simulink model "long"  (R2013b)
settings: Solver=ode45  StartTime=0.0  StopTime=10  RelTol=1e-3
values from neighbouring files (symbols this model uses):
  A = [[X_u, X_w, 0, -g*cos(theta_0), 0] ... (first row only)    [hw3.m]
  B = [X_d_e ... (first row only)    [hw3.m]
  C = eye(5)    [hw3.m]
  D = [0; 0; 0; 0; 0]    [hw3.m]
libraries: simulink_extras x6
settings Model: Creator=rjoyce  LastModifiedBy=Johnny
settings DataIOCC: SignalLoggingSaveFormat=ModelDataLogs
settings OptimizationCC: ExpressionDepthLimit=2147483647  SimCompilerOptimization=off
settings DebuggingCC: FcnCallInpInsideContextMsg=UseLocalSettings  FrameProcessingCompatibilityMsg=error  StateNameClashWarn=warning
settings RTWCC: RTWCompilerOptimization=off
settings GRTTargetCC: TargetLangStandard=C89/C90 (ANSI)  CodeReplacementLibrary=None  CombineOutputUpdateFcns=off  CPPClassGenCompliant=on  GRTInterface=on

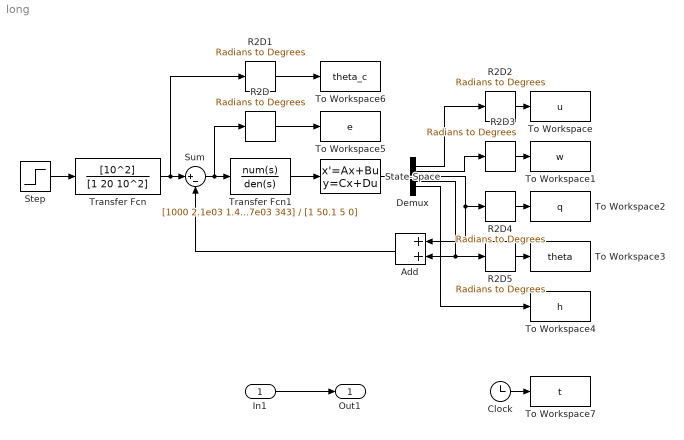
== system long ==
  In1 : Inport
  Add : Sum
  Clock : Clock
  Demux : Demux  Outputs=5
  R2D{,1..5} (6 alike) : simulink_extras/Transformations/Radians to Degrees
  State-Space : StateSpace  A=A  B=B  C=C  D=D  X0=[0 0 0 0 0]
  Step : Step  Time=0  After=5/57.3  SampleTime=0
  Sum : Sum  Inputs=|+-
  To Workspace : ToWorkspace  VariableName=u  SampleTime=-1
  To Workspace1 : ToWorkspace  VariableName=w  SampleTime=-1
  To Workspace2 : ToWorkspace  VariableName=q  SampleTime=-1
  To Workspace3 : ToWorkspace  VariableName=theta  SampleTime=-1
  To Workspace4 : ToWorkspace  VariableName=h  SampleTime=-1
  To Workspace5 : ToWorkspace  VariableName=e  SampleTime=-1
  To Workspace6 : ToWorkspace  VariableName=theta_c  SampleTime=-1
  To Workspace7 : ToWorkspace  VariableName=t  SampleTime=-1
  Transfer Fcn : TransferFcn  Numerator=[10^2]  Denominator=[1 20 10^2]
  Transfer Fcn1 : TransferFcn  Numerator=[1000 2.1e03 1.47e03 343]  Denominator=[1 50.1 5 0]
  Out1 : Outport
  wires:
  State-Space/1 -> Demux/1
  Demux/1 -> R2D2/1
  Demux/2 -> R2D3/1
  Demux/3 -> R2D4/1, Add/1
  Demux/4 -> R2D5/1, Add/2
  Transfer Fcn/1 -> Sum/1, R2D1/1
  Step/1 -> Transfer Fcn/1
  Sum/1 -> R2D/1, Transfer Fcn1/1
  Add/1 -> Sum/2
  R2D/1 -> To Workspace5/1
  R2D1/1 -> To Workspace6/1
  R2D2/1 -> To Workspace/1
  R2D3/1 -> To Workspace1/1
  R2D4/1 -> To Workspace2/1
  R2D5/1 -> To Workspace3/1
  Demux/5 -> To Workspace4/1
  Clock/1 -> To Workspace7/1
  Transfer Fcn1/1 -> State-Space/1
  In1/1 -> Out1/1
